simulink model "pressingswitch_fan_experiment"  (R2021a)
settings: Solver=FixedStepAuto  StartTime=0.0  StopTime=11  FixedStep=0.01  RelTol=1e-3
libraries: simulink x1
settings Model: Creator=surya  LastModifiedBy=surya

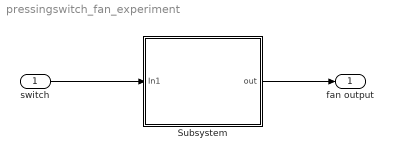
== system pressingswitch_fan_experiment ==
  switch : Inport
  Subsystem : Subsystem
  fan output : Outport
  wires:
  switch/1 -> Subsystem/1(In1)
  Subsystem/1(out) -> fan output/1

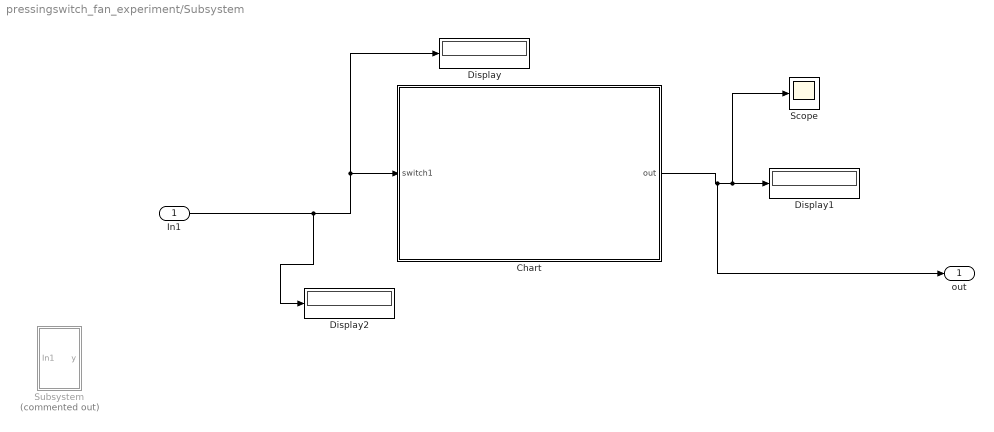
== system pressingswitch_fan_experiment/Subsystem ==
  In1 : Inport
  Chart : Stateflow chart  TreatAsAtomicUnit=on
  Display : Display
  Display1 : Display
  Display2 : Display
  Scope : Scope
  Subsystem : Subsystem  Commented=on
  out : Outport
  wires:
  Chart/1(out) -> out/1, Scope/1, Display1/1
  In1/1 -> Display2/1, Display/1, Chart/1(switch1)

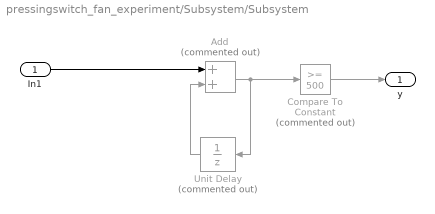
== system pressingswitch_fan_experiment/Subsystem/Subsystem ==
  In1 : Inport
  Add : Sum  Commented=on
  Compare To Constant : simulink/Logic and Bit Operations/Compare To Constant  Commented=on  relop=>=  const=500  OutDataTypeStr=boolean
  Unit Delay : UnitDelay  Commented=on  SampleTime=-1  HasFrameUpgradeWarning=on
  y : Outport
  wires:
  Add/1 -> Unit Delay/1, Compare To Constant/1
  Unit Delay/1 -> Add/2
  Compare To Constant/1 -> y/1
  In1/1 -> Add/1

== stateflow chart pressingswitch_fan_experiment/Subsystem/Chart ==
  state FANlogic
    state timer1=timerr(t) [function]
      (default) -> (junction 22) : % Timer
      (junction 22) -> (junction 24) : {timer1=t}
      (junction 24) -> (junction 23) [order 1] : [switch1==1 & timer1>=500]
      (junction 25) -> (junction 24)
      (junction 23) -> (junction 25) : {timer1 = timer1 + 1;}
      (junction 24) -> (junction 26) [order 2]
    state OFF
      en: out=0;
    state ON
      en:out=1;
    (default) -> OFF
    OFF -> ON : [timerr(0)>=500 & switch1==1&after(10,sec)]
    ON -> OFF : [ switch1==0]
  data: timer1 function_output; t function_input; switch1 input; out output; timer local; timer1 local
